simulink library "InverseK_Lib"  (R2014a)
settings: Solver=ode45  StartTime=0.0  StopTime=10  RelTol=1e-3
settings Model: Creator=Cat  LastModifiedBy=Cat

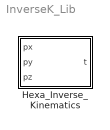
== system InverseK_Lib ==
  Hexa_Inverse_Kinematics : MATLAB Function  TreatAsAtomicUnit=on

== matlab function InverseK_Lib/Hexa_Inverse_Kinematics ==
  data: px input; t output; py input; pz input
function t = Hexa_Inverse_Kinematics(px,py,pz)
%#codegen

%    This function was generated by the Symbolic Math Toolbox version 6.0.
%    29-Sep-2015 02:51:47

t2 = sqrt(3.0);
t3 = px.*-5.0e-1i;
t4 = py.*(1.0./2.0);
t5 = px.*t2.*(1.0./2.0);
t6 = py.*t2.*5.0e-1i;
t7 = t3+t4+t5+t6-4.0./5.0;
t10 = px.*(1.0./2.0);
t11 = py.*t2.*(1.0./2.0);
t8 = t10-t11;
t9 = abs(t7);
t12 = t8.^2;
t13 = 1.0./t9;
t14 = t4+t5-4.0./5.0;
t15 = 1.0./t9.^2;
t16 = t14.^2;
t18 = t12.*t13;
t19 = t12.*t15.*(4.0./5.0);
t20 = t13.*t16;
t21 = t15.*t16.*(4.0./5.0);
t17 = t18-t19+t20-t21;
t22 = t17.^2;
t23 = pz.^2;
t24 = t22+t23;
t25 = sign(t24);
t26 = sqrt(t25);
t28 = t22.*(2.5e1./3.2e1);
t29 = t23.*(2.5e1./3.2e1);
t27 = t28+t29-1.0;
t = [angle(t7),-angle(sqrt(t22.*(-2.5e1./6.4e1)-t23.*(2.5e1./6.4e1)+1.0).*1.6i+sqrt(t24))-pi.*t26.*(t26-1.0).*(1.0./2.0),angle(t28+t29-sqrt(-t27.^2+1.0).*1i-1.0)];
